simulink library "pms"  (R2013a)
settings: Solver=ode45  StartTime=0.0  StopTime=10.0  RelTol=1e-3
undefined symbols (not defined in the file): engines, flrRampTime, flrRestoreTime, nBatteries, nSwitchboard, nThrusters, PMSenableFaultDetection, pmsSamplingTime, powerDesiredDPBias, powerDesiredDPGain, rampTimePowerAvaialble, rampTimeUpload, reactionTimePowerAvaialble, vNL0, wNL0
libraries: pms x1
settings Model: Creator=torstein  LastModifiedBy=torstebo

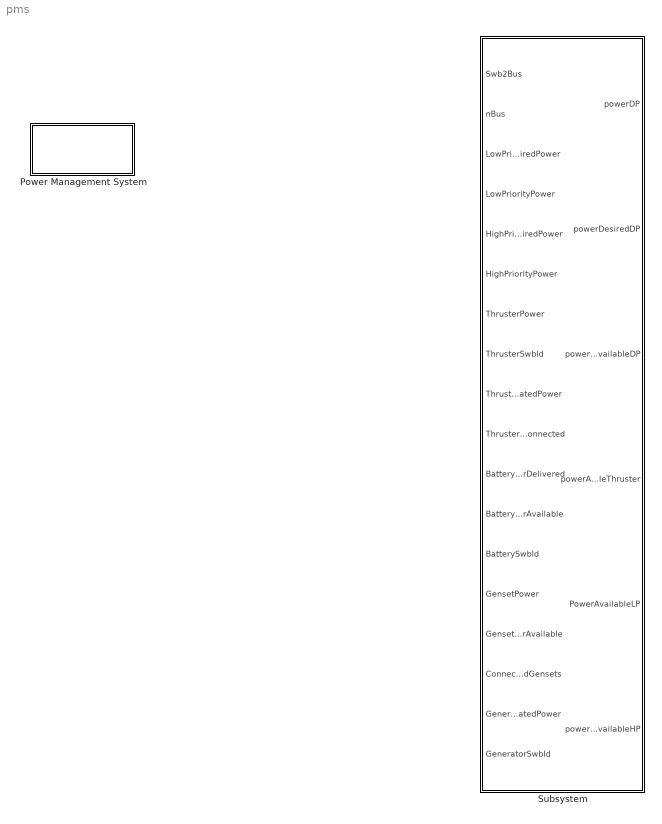
== system pms ==
  Power Management System : Subsystem  Tag=PowerManagementSystem
  Subsystem : Subsystem  mask{TSample=pmsSamplingTime, reactionTimePowerAvaialble=reactionTimePowerAvaialble, rampTimePowerAvaialble=rampTimePowerAvaialble, FlrRestoreTime=flrRestoreTime, FlrRampTime=flrRampTime, nSwb=nSwitchboard, nThruster=nThrusters, nBatteries=nBatteries, DPPowerAvailableBias=powerDesiredDPBias, DPPowerAvailableGain=powerDesiredDPGain, PMSenableFaultDetection=PMSenableFaultDetection}
      mask prompts: TSample "Sampling time (-1 if continous)"; reactionTimePowerAvaialble "Reaction time power available"; rampTimePowerAvaialble "Ramp time power available"; FlrRestoreTime "Fast load reduction restore time"; FlrRampTime "Fast load reduction ramp time"; nSwb "Number of switchboards"; nThruster "Number of thrusters"; nBatteries "Number of emergency batteries"; DPPowerAvailableBias "Power available bias for DP in % of rated power of thrusters"; DPPowerAvailableGain "Power available gain for DP (power available DP = powerThrusters*gain+bias)"; PMSenableFaultDetection "Enable fault detection"

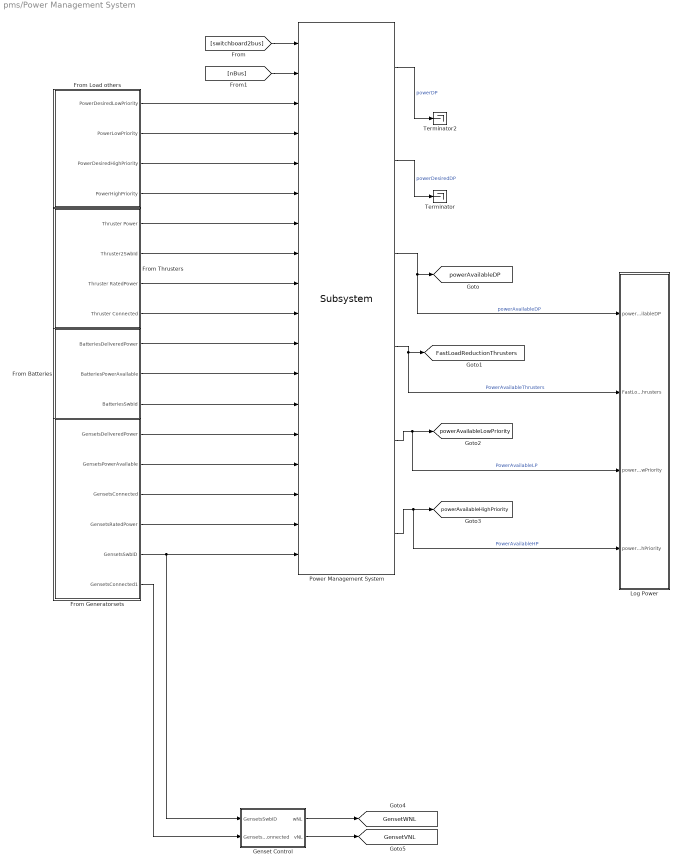
== system pms/Power Management System ==
  From Batteries : Subsystem  Tag=PowerManagementSystem/FromBatteries
  From Generatorsets : Subsystem  Tag=PowerManagementSystem/FromGeneratorset
  From Load others : Subsystem  Tag=PowerManagementSystem/LoadOthersFrom
  From Thrusters : Subsystem  Tag=PowerManagementSystem/ThrusterFrom
  Genset Control : Subsystem
  Log Power : Subsystem
  Power Management System : pms/Subsystem  TSample=pmsSamplingTime  reactionTimePowerAvaialble=reactionTimePowerAvaialble  rampTimePowerAvaialble=rampTimePowerAvaialble  FlrRestoreTime=flrRestoreTime  FlrRampTime=flrRampTime  nSwb=nSwitchboard  nThruster=nThrusters  nBatteries=nBatteries  DPPowerAvailableBias=powerDesiredDPBias  DPPowerAvailableGain=powerDesiredDPGain  PMSenableFaultDetection=PMSenableFaultDetection
  Terminator : Terminator
  Terminator2 : Terminator
  tag scope: FastLoadReductionThrusters=global, GensetVNL=global, GensetWNL=global, powerAvailableDP=global, powerAvailableHighPriority=global, powerAvailableLowPriority=global
  wires:
  Power Management System/4 -> Log Power/2(FastLoadReductionThrusters), [FastLoadReductionThrusters]  "PowerAvailableThrusters"
  Power Management System/6 -> Log Power/4(powerAvailableHighPriority), [powerAvailableHighPriority]  "PowerAvailableHP"
  Power Management System/3 -> Log Power/1(powerAvailableDP), [powerAvailableDP]  "powerAvailableDP"
  Power Management System/5 -> Log Power/3(powerAvailableLowPriority), [powerAvailableLowPriority]  "PowerAvailableLP"
  [nBus] -> Power Management System/2
  Power Management System/1 -> Terminator2/1  "powerDP"
  Power Management System/2 -> Terminator/1  "powerDesiredDP"
  [switchboard2bus] -> Power Management System/1
  From Load others/1(PowerDesiredLowPriority) -> Power Management System/3
  From Load others/3(PowerDesiredHighPriority) -> Power Management System/5
  From Load others/2(PowerLowPriority) -> Power Management System/4
  From Load others/4(PowerHighPriority) -> Power Management System/6
  From Thrusters/1(Thruster Power) -> Power Management System/7
  From Thrusters/2(Thruster2SwbId) -> Power Management System/8
  From Thrusters/3(Thruster RatedPower) -> Power Management System/9
  From Thrusters/4(Thruster Connected) -> Power Management System/10
  From Generatorsets/1(GensetsDeliveredPower) -> Power Management System/14
  From Generatorsets/2(GensetsPowerAvailable) -> Power Management System/15
  From Generatorsets/4(GensetsRatedPower) -> Power Management System/17
  Genset Control/1(wNL) -> [GensetWNL]
  From Generatorsets/3(GensetsConnected) -> Power Management System/16
  From Generatorsets/5(GensetsSwbID) -> Genset Control/1(GensetsSwbID), Power Management System/18
  From Generatorsets/6(GensetsConnected1) -> Genset Control/2(GensetsConnected)
  Genset Control/2(vNL) -> [GensetVNL]
  From Batteries/3(BatteriesSwbId) -> Power Management System/13
  From Batteries/2(BatteriesPowerAvailable) -> Power Management System/12
  From Batteries/1(BatteriesDeliveredPower) -> Power Management System/11

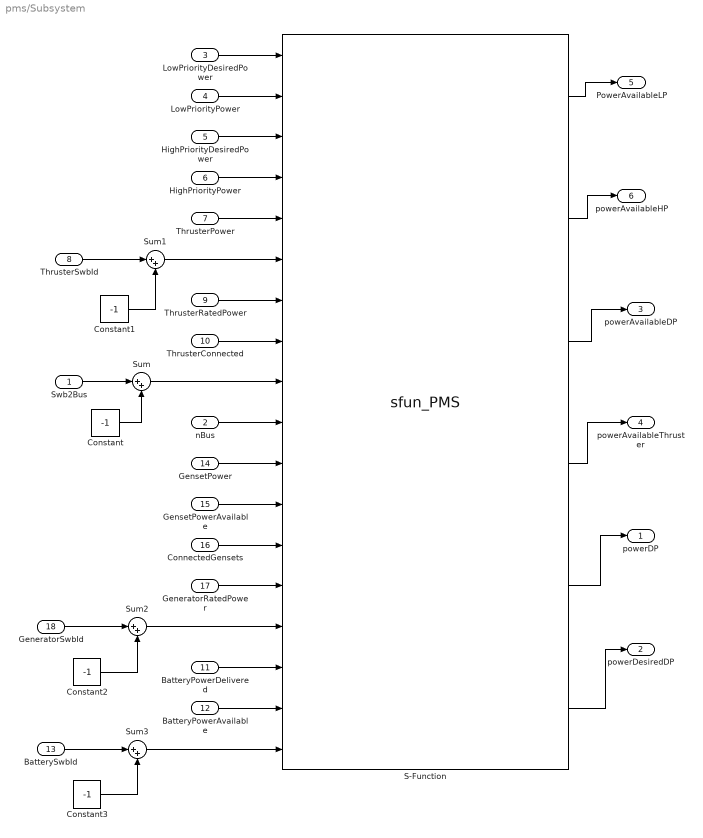
== system pms/Subsystem ==
  Swb2Bus : Inport
  nBus : Inport  Port=2
  LowPriorityDesiredPower : Inport  Port=3
  LowPriorityPower : Inport  Port=4
  HighPriorityDesiredPower : Inport  Port=5
  HighPriorityPower : Inport  Port=6
  ThrusterPower : Inport  Port=7
  ThrusterSwbId : Inport  Port=8
  ThrusterRatedPower : Inport  Port=9
  ThrusterConnected : Inport  Port=10
  BatteryPowerDelivered : Inport  Port=11
  BatteryPowerAvailable : Inport  Port=12
  BatterySwbId : Inport  Port=13
  GensetPower : Inport  Port=14
  GensetPowerAvailable : Inport  Port=15
  ConnectedGensets : Inport  Port=16
  GeneratorRatedPower : Inport  Port=17
  GeneratorSwbId : Inport  Port=18
  Constant{,1..3} (4 alike) : Constant  Value=-1
  S-Function : S-Function  FunctionName=sfun_PMS  Parameters=TSample, reactionTimePowerAvaialble, rampTimePowerAvaialble,FlrRestoreTime,FlrRampTime,nSwb,nThruster,nBatteries,DPPowerAvailableBias,DPPowerAvailableGain,PMSenableFaultDetection  EnableBusSupport=off
  Sum{,1..3} (4 alike) : Sum  Inputs=|++
  powerDP : Outport
  powerDesiredDP : Outport  Port=2
  powerAvailableDP : Outport  Port=3
  powerAvailableThruster : Outport  Port=4
  PowerAvailableLP : Outport  Port=5
  powerAvailableHP : Outport  Port=6
  wires:
  Sum3/1 -> S-Function/18
  BatterySwbId/1 -> Sum3/1
  Constant3/1 -> Sum3/2
  BatteryPowerAvailable/1 -> S-Function/17
  BatteryPowerDelivered/1 -> S-Function/16
  S-Function/6 -> powerDesiredDP/1
  S-Function/5 -> powerDP/1
  Sum2/1 -> S-Function/15
  GeneratorRatedPower/1 -> S-Function/14
  ConnectedGensets/1 -> S-Function/13
  GensetPowerAvailable/1 -> S-Function/12
  GensetPower/1 -> S-Function/11
  nBus/1 -> S-Function/10
  Sum/1 -> S-Function/9
  ThrusterConnected/1 -> S-Function/8
  ThrusterRatedPower/1 -> S-Function/7
  Sum1/1 -> S-Function/6
  GeneratorSwbId/1 -> Sum2/1
  Constant2/1 -> Sum2/2
  Constant1/1 -> Sum1/2
  ThrusterSwbId/1 -> Sum1/1
  Swb2Bus/1 -> Sum/1
  Constant/1 -> Sum/2
  ThrusterPower/1 -> S-Function/5
  S-Function/3 -> powerAvailableDP/1
  HighPriorityPower/1 -> S-Function/4
  S-Function/1 -> PowerAvailableLP/1
  LowPriorityDesiredPower/1 -> S-Function/1
  HighPriorityDesiredPower/1 -> S-Function/3
  LowPriorityPower/1 -> S-Function/2
  S-Function/2 -> powerAvailableHP/1
  S-Function/4 -> powerAvailableThruster/1

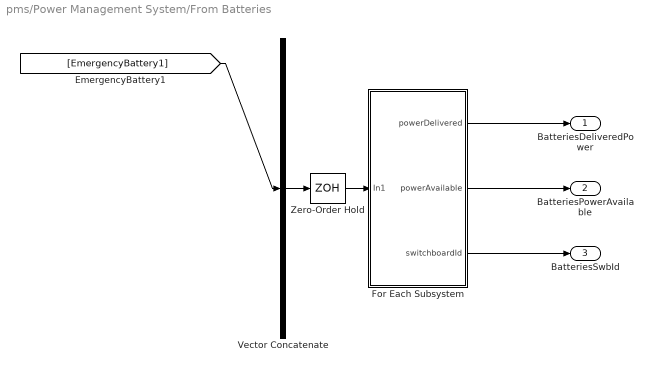
== system pms/Power Management System/From Batteries ==
  For Each Subsystem : Subsystem  TreatAsAtomicUnit=on
  Vector Concatenate : Concatenate  Tag=PowerManagementSystem/FromBatteries/Merger  NumInputs=1
  Zero-Order Hold : ZeroOrderHold  SampleTime=pmsSamplingTime
  BatteriesDeliveredPower : Outport
  BatteriesPowerAvailable : Outport  Port=2
  BatteriesSwbId : Outport  Port=3
  wires:
  For Each Subsystem/3(switchboardId) -> BatteriesSwbId/1
  For Each Subsystem/2(powerAvailable) -> BatteriesPowerAvailable/1
  For Each Subsystem/1(powerDelivered) -> BatteriesDeliveredPower/1
  Vector Concatenate/1 -> Zero-Order Hold/1
  Zero-Order Hold/1 -> For Each Subsystem/1(In1)
  [EmergencyBattery1] -> Vector Concatenate/1

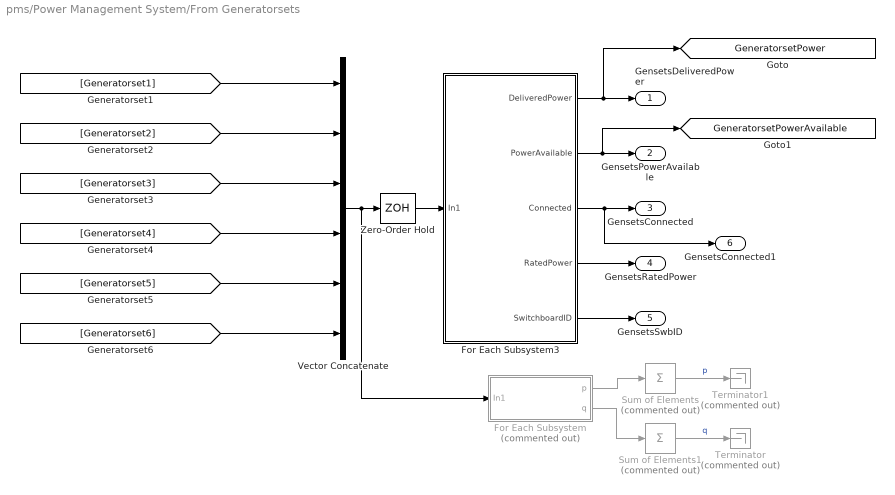
== system pms/Power Management System/From Generatorsets ==
  For Each Subsystem : Subsystem  Commented=on  TreatAsAtomicUnit=on
  For Each Subsystem3 : Subsystem  TreatAsAtomicUnit=on
  Sum of Elements : Sum  Commented=on  Inputs=+
  Sum of Elements1 : Sum  Commented=on  Inputs=+
  Terminator : Terminator  Commented=on
  Terminator1 : Terminator  Commented=on
  Vector Concatenate : Concatenate  Tag=PowerManagementSystem/FromGeneratorset/Merger  NumInputs=6
  Zero-Order Hold : ZeroOrderHold  SampleTime=pmsSamplingTime
  GensetsDeliveredPower : Outport  OutDataTypeStr=double
  GensetsPowerAvailable : Outport  Port=2  OutDataTypeStr=double
  GensetsConnected : Outport  Port=3  OutDataTypeStr=boolean
  GensetsRatedPower : Outport  Port=4  OutDataTypeStr=double
  GensetsSwbID : Outport  Port=5  OutDataTypeStr=uint8
  GensetsConnected1 : Outport  Port=6  OutDataTypeStr=boolean
  tag scope: GeneratorsetPower=global, GeneratorsetPowerAvailable=global
  wires:
  For Each Subsystem3/3(Connected) -> GensetsConnected1/1, GensetsConnected/1
  For Each Subsystem3/5(SwitchboardID) -> GensetsSwbID/1
  For Each Subsystem3/2(PowerAvailable) -> [GeneratorsetPowerAvailable], GensetsPowerAvailable/1
  For Each Subsystem3/4(RatedPower) -> GensetsRatedPower/1
  For Each Subsystem3/1(DeliveredPower) -> [GeneratorsetPower], GensetsDeliveredPower/1
  Vector Concatenate/1 -> Zero-Order Hold/1, For Each Subsystem/1(In1)
  For Each Subsystem/1(p) -> Sum of Elements/1
  For Each Subsystem/2(q) -> Sum of Elements1/1
  Sum of Elements1/1 -> Terminator/1  "q"
  Sum of Elements/1 -> Terminator1/1  "p"
  Zero-Order Hold/1 -> For Each Subsystem3/1(In1)
  [Generatorset1] -> Vector Concatenate/1
  [Generatorset2] -> Vector Concatenate/2
  [Generatorset6] -> Vector Concatenate/6
  [Generatorset3] -> Vector Concatenate/3
  [Generatorset4] -> Vector Concatenate/4
  [Generatorset5] -> Vector Concatenate/5

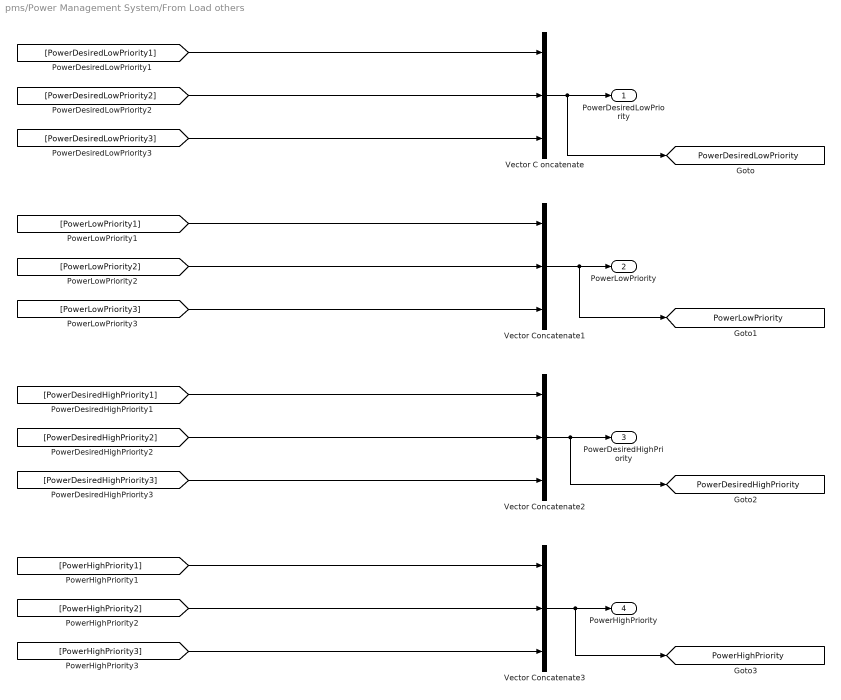
== system pms/Power Management System/From Load others ==
  Vector C oncatenate : Concatenate  Tag=PowerManagementSystem/LoadOthersFrom/PowerDesiredLowPriority  NumInputs=3
  Vector Concatenate1 : Concatenate  Tag=PowerManagementSystem/LoadOthersFrom/PowerLowPriority  NumInputs=3
  Vector Concatenate2 : Concatenate  Tag=PowerManagementSystem/LoadOthersFrom/PowerDesiredHighPriority  NumInputs=3
  Vector Concatenate3 : Concatenate  Tag=PowerManagementSystem/LoadOthersFrom/PowerHighPriority  NumInputs=3
  PowerDesiredLowPriority : Outport
  PowerLowPriority : Outport  Port=2
  PowerDesiredHighPriority : Outport  Port=3
  PowerHighPriority : Outport  Port=4
  tag scope: PowerDesiredHighPriority=global, PowerDesiredLowPriority=global, PowerHighPriority=global, PowerLowPriority=global
  wires:
  Vector C oncatenate/1 -> PowerDesiredLowPriority/1, [PowerDesiredLowPriority]
  Vector Concatenate1/1 -> [PowerLowPriority], PowerLowPriority/1
  Vector Concatenate2/1 -> [PowerDesiredHighPriority], PowerDesiredHighPriority/1
  Vector Concatenate3/1 -> [PowerHighPriority], PowerHighPriority/1
  [PowerDesiredLowPriority1] -> Vector C oncatenate/1
  [PowerLowPriority1] -> Vector Concatenate1/1
  [PowerDesiredHighPriority1] -> Vector Concatenate2/1
  [PowerHighPriority1] -> Vector Concatenate3/1
  [PowerDesiredLowPriority2] -> Vector C oncatenate/2
  [PowerLowPriority2] -> Vector Concatenate1/2
  [PowerDesiredHighPriority2] -> Vector Concatenate2/2
  [PowerHighPriority2] -> Vector Concatenate3/2
  [PowerDesiredLowPriority3] -> Vector C oncatenate/3
  [PowerLowPriority3] -> Vector Concatenate1/3
  [PowerDesiredHighPriority3] -> Vector Concatenate2/3
  [PowerHighPriority3] -> Vector Concatenate3/3

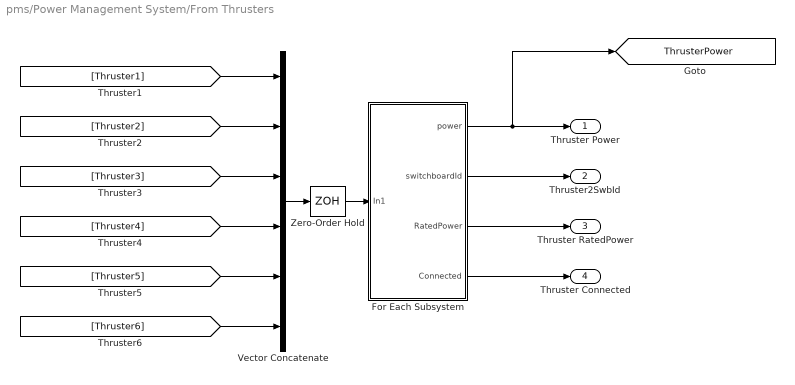
== system pms/Power Management System/From Thrusters ==
  For Each Subsystem : Subsystem  TreatAsAtomicUnit=on
  Vector Concatenate : Concatenate  Tag=FromThrusters/Merger  NumInputs=6
  Zero-Order Hold : ZeroOrderHold  SampleTime=pmsSamplingTime
  Thruster Power : Outport
  Thruster2SwbId : Outport  Port=2
  Thruster RatedPower : Outport  Port=3
  Thruster Connected : Outport  Port=4
  tag scope: ThrusterPower=global
  wires:
  For Each Subsystem/3(RatedPower) -> Thruster RatedPower/1
  For Each Subsystem/2(switchboardId) -> Thruster2SwbId/1
  For Each Subsystem/1(power) -> [ThrusterPower], Thruster Power/1
  For Each Subsystem/4(Connected) -> Thruster Connected/1
  Vector Concatenate/1 -> Zero-Order Hold/1
  Zero-Order Hold/1 -> For Each Subsystem/1(In1)
  [Thruster1] -> Vector Concatenate/1
  [Thruster2] -> Vector Concatenate/2
  [Thruster3] -> Vector Concatenate/3
  [Thruster4] -> Vector Concatenate/4
  [Thruster5] -> Vector Concatenate/5
  [Thruster6] -> Vector Concatenate/6

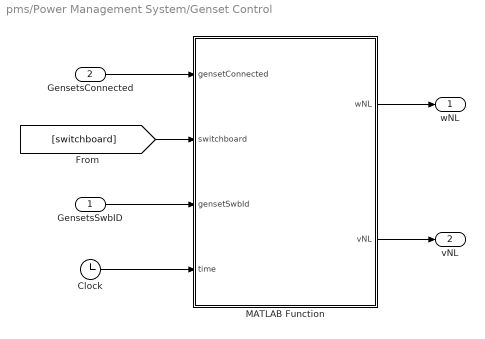
== system pms/Power Management System/Genset Control ==
  GensetsSwbID : Inport
  GensetsConnected : Inport  Port=2
  Clock : Clock
  MATLAB Function : MATLAB Function  TreatAsAtomicUnit=on
  wNL : Outport
  vNL : Outport  Port=2
  wires:
  MATLAB Function/1(wNL) -> wNL/1
  [switchboard] -> MATLAB Function/2(switchboard)
  GensetsConnected/1 -> MATLAB Function/1(gensetConnected)
  GensetsSwbID/1 -> MATLAB Function/3(gensetSwbId)
  Clock/1 -> MATLAB Function/4(time)
  MATLAB Function/2(vNL) -> vNL/1

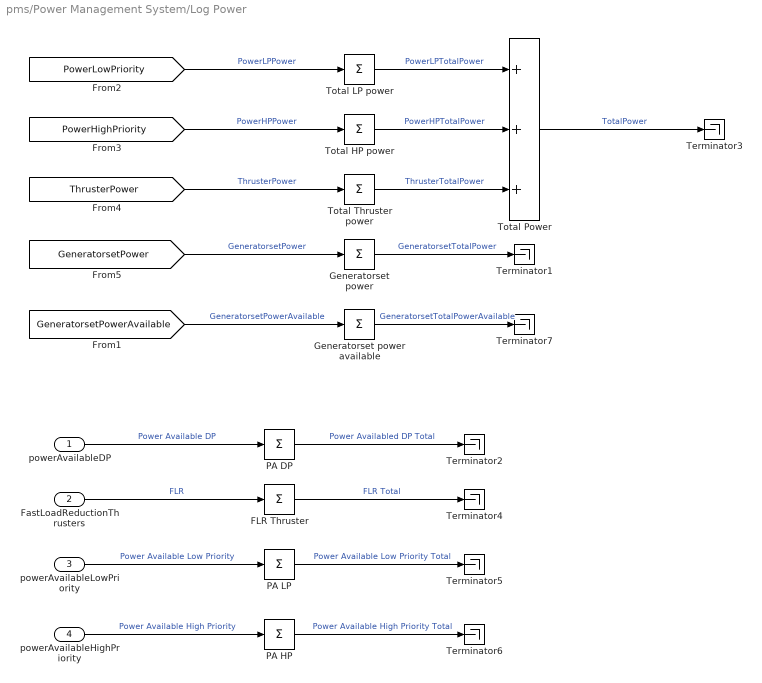
== system pms/Power Management System/Log Power ==
  powerAvailableDP : Inport
  FastLoadReductionThrusters : Inport  Port=2
  powerAvailableLowPriority : Inport  Port=3
  powerAvailableHighPriority : Inport  Port=4
  FLR Thruster : Sum  Inputs=+
  Generatorset power : Sum  Inputs=+
  Generatorset power available : Sum  Inputs=+
  PA DP : Sum  Inputs=+
  PA HP : Sum  Inputs=+
  PA LP : Sum  Inputs=+
  Terminator{1..7} (7 alike) : Terminator
  Total HP power : Sum  Inputs=+
  Total LP power : Sum  Inputs=+
  Total Power : Sum  Inputs=3
  Total Thruster power : Sum  Inputs=+
  wires:
  [PowerHighPriority] -> Total HP power/1  "PowerHPPower"
  Total HP power/1 -> Total Power/2  "PowerHPTotalPower"
  Total Power/1 -> Terminator3/1  "TotalPower"
  Generatorset power/1 -> Terminator1/1  "GeneratorsetTotalPower"
  [GeneratorsetPower] -> Generatorset power/1  "GeneratorsetPower"
  [ThrusterPower] -> Total Thruster power/1  "ThrusterPower"
  Total Thruster power/1 -> Total Power/3  "ThrusterTotalPower"
  Total LP power/1 -> Total Power/1  "PowerLPTotalPower"
  [PowerLowPriority] -> Total LP power/1  "PowerLPPower"
  powerAvailableDP/1 -> PA DP/1  "Power Available DP"
  PA DP/1 -> Terminator2/1  "Power Availabled DP Total"
  FastLoadReductionThrusters/1 -> FLR Thruster/1  "FLR"
  FLR Thruster/1 -> Terminator4/1  "FLR Total"
  powerAvailableLowPriority/1 -> PA LP/1  "Power Available Low Priority"
  powerAvailableHighPriority/1 -> PA HP/1  "Power Available High Priority"
  PA LP/1 -> Terminator5/1  "Power Available Low Priority Total"
  PA HP/1 -> Terminator6/1  "Power Available High Priority Total"
  Generatorset power available/1 -> Terminator7/1  "GeneratorsetTotalPowerAvailable"
  [GeneratorsetPowerAvailable] -> Generatorset power available/1  "GeneratorsetPowerAvailable"

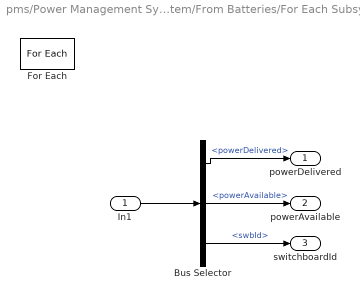
== system pms/Power Management System/From Batteries/For Each Subsystem ==
  In1 : Inport  Partition=on  PartitionDimension=1  PartitionWidth=1
  Bus Selector : BusSelector  OutputSignals=powerDelivered,powerAvailable,swbId
  For Each : ForEach  DisableCoverage=on  IndexMode=One-based
  powerDelivered : Outport  OutDataTypeStr=double  ConcatenationDimension=1
  powerAvailable : Outport  Port=2  OutDataTypeStr=double  ConcatenationDimension=1
  switchboardId : Outport  Port=3  OutDataTypeStr=uint8  ConcatenationDimension=1
  wires:
  In1/1 -> Bus Selector/1
  Bus Selector/1 -> powerDelivered/1  "<powerDelivered>"
  Bus Selector/2 -> powerAvailable/1  "<powerAvailable>"
  Bus Selector/3 -> switchboardId/1  "<swbId>"

== system pms/Power Management System/From Generatorsets/For Each Subsystem ==
  In1 : Inport  Partition=on  PartitionDimension=1  PartitionWidth=1
  Bus Selector : BusSelector  OutputSignals=P,Q
  For Each : ForEach  DisableCoverage=on  IndexMode=One-based
  p : Outport  ConcatenationDimension=1
  q : Outport  Port=2  ConcatenationDimension=1
  wires:
  In1/1 -> Bus Selector/1
  Bus Selector/1 -> p/1  "<P>"
  Bus Selector/2 -> q/1  "<Q>"

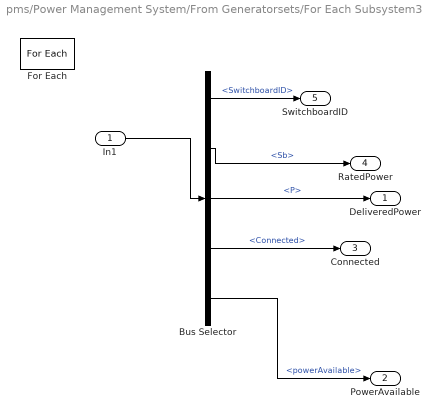
== system pms/Power Management System/From Generatorsets/For Each Subsystem3 ==
  In1 : Inport  OutDataTypeStr=Bus: Genset2PMS  Partition=on  PartitionDimension=1  PartitionWidth=1
  Bus Selector : BusSelector  OutputSignals=SwitchboardID,Sb,P,Connected,powerAvailable
  For Each : ForEach  DisableCoverage=on  IndexMode=One-based
  DeliveredPower : Outport  OutDataTypeStr=double  ConcatenationDimension=1
  PowerAvailable : Outport  Port=2  OutDataTypeStr=double  ConcatenationDimension=1
  Connected : Outport  Port=3  OutDataTypeStr=boolean  ConcatenationDimension=1
  RatedPower : Outport  Port=4  OutDataTypeStr=double  ConcatenationDimension=1
  SwitchboardID : Outport  Port=5  OutDataTypeStr=uint8  ConcatenationDimension=1
  wires:
  In1/1 -> Bus Selector/1
  Bus Selector/2 -> RatedPower/1  "<Sb>"
  Bus Selector/1 -> SwitchboardID/1  "<SwitchboardID>"
  Bus Selector/3 -> DeliveredPower/1  "<P>"
  Bus Selector/4 -> Connected/1  "<Connected>"
  Bus Selector/5 -> PowerAvailable/1  "<powerAvailable>"

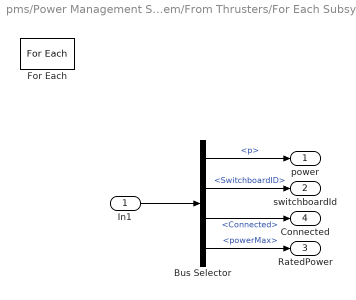
== system pms/Power Management System/From Thrusters/For Each Subsystem ==
  In1 : Inport  OutDataTypeStr=Bus: ThrusterBus  Partition=on  PartitionDimension=1  PartitionWidth=1
  Bus Selector : BusSelector  OutputSignals=power.p,SwitchboardID,Connected,powerMax
  For Each : ForEach  DisableCoverage=on  IndexMode=One-based
  power : Outport  OutDataTypeStr=double  ConcatenationDimension=1
  switchboardId : Outport  Port=2  OutDataTypeStr=uint8  ConcatenationDimension=1
  RatedPower : Outport  Port=3  OutDataTypeStr=double  ConcatenationDimension=1
  Connected : Outport  Port=4  OutDataTypeStr=boolean  ConcatenationDimension=1
  wires:
  In1/1 -> Bus Selector/1
  Bus Selector/1 -> power/1  "<p>"
  Bus Selector/2 -> switchboardId/1  "<SwitchboardID>"
  Bus Selector/3 -> Connected/1  "<Connected>"
  Bus Selector/4 -> RatedPower/1  "<powerMax>"

== matlab function pms/Power Management System/Genset Control/MATLAB Function ==
  data: wNL0 parameter; vNL0 parameter; wNL output double; engines parameter; gensetConnected input; switchboard input; gensetSwbId input; time input; rampTimeUpload parameter; vNL output
function [wNL, vNL] = loadSharingControl(wNL0,vNL0,engines,gensetConnected,switchboard,gensetSwbId,time,rampTimeUpload)
wNL = ones(engines,1);
vNL = ones(engines,1);
persistent timeConnected;
if isempty(timeConnected)
    timeConnected = -inf*ones(engines,1);
end

for i = 1:engines
    if (gensetConnected(i))
        if (timeConnected(i)+rampTimeUpload<=time)
            wNL(i) = wNL0(i);
            vNL(i) = vNL0(i);
        else
            a = (time-timeConnected(i))/rampTimeUpload;
            wNL(i) = wNL0(i)*a+switchboard(gensetSwbId(i)).omega*(1-a);
            vNL(i) = vNL0(i)*a+abs(switchboard(gensetSwbId(i)).voltage)*(1-a);
    
        end
    else
        timeConnected(i) = time;
        wNL(i) = switchboard(gensetSwbId(i)).omega;
        vNL(i) = abs(switchboard(gensetSwbId(i)).voltage);
    end
end
